simulink model "demo3c"  (Simulink 7.4)
settings: Solver=ode3  StartTime=0.0  StopTime=4  MinStep=0.000  RelTol=1e-3
undefined symbols (not defined in the file): disturb, fgamma, lambda11, lambda12, lambda21, lambda22, Mdisturb
libraries: roblocks x3, simulink x1
settings Model: Creator=pic  LastModifiedBy=acolome  ExtModeTrigMode=oneshot  ExtModeArmWhenConnect=off
settings DataIOCC: LimitDataPoints=off
settings OptimizationCC: BlockReduction=off  BooleanDataType=off  InitFltsAndDblsToZero=on
settings DebuggingCC: SaveWithParameterizedLinksMsg=none  SignalResolutionControl=TryResolveAllWithWarning  SolverPrmCheckMsg=none  MultiTaskDSMMsg=warning  MultiTaskCondExecSysMsg=none  StrictBusMsg=None
settings HardwareCC: TargetUnknown=on
settings RTWCC: IncludeERTFirstTime=on
settings GRTTargetCC: ModelReferenceCompliant=off  ParMdlRefBuildCompliant=off  CompOptLevelCompliant=off  MatFileLogging=off

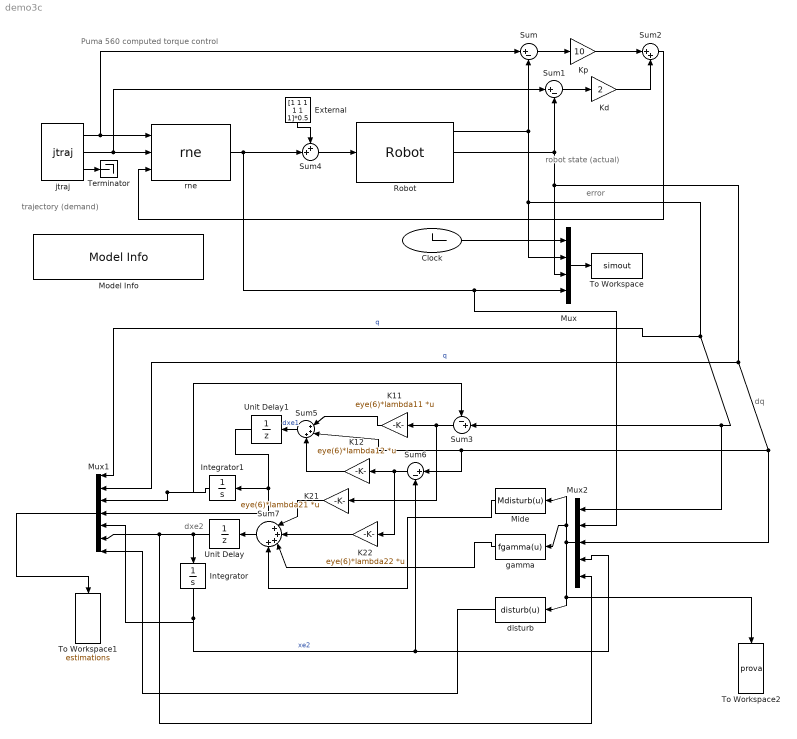
== system demo3c ==
  note: Puma 560 computed torque control
  note: trajectory
      | (demand)
  note: robot state
      | (actual)
  note: error
  note: dq
  note: dxe2
  Clock : Clock
      settings: Decimation=100
  External : Constant  Value=[1 1 1 1 1 1]*0.5  OutDataType=fixdt(1, 16)  OutScaling=2^0
  Integrator : Integrator
  Integrator1 : Integrator
  K11 : Gain  Gain=eye(6)*lambda11  Multiplication=Matrix(K*u)  ParameterDataType=fixdt(1, 16)  ParameterScaling=2^0  OutDataType=fixdt(1, 16)  OutScaling=2^0
  K12 : Gain  Gain=eye(6)*lambda12  Multiplication=Matrix(K*u)  ParameterDataType=fixdt(1, 16)  ParameterScaling=2^0  OutDataType=fixdt(1, 16)  OutScaling=2^0
  K21 : Gain  Gain=eye(6)*lambda21  Multiplication=Matrix(K*u)  ParameterDataType=fixdt(1, 16)  ParameterScaling=2^0  OutDataType=fixdt(1, 16)  OutScaling=2^0
  K22 : Gain  Gain=eye(6)*lambda22  Multiplication=Matrix(K*u)  ParameterDataType=fixdt(1, 16)  ParameterScaling=2^0  OutDataType=fixdt(1, 16)  OutScaling=2^0
  Kd : Gain  Gain=2  SaturateOnIntegerOverflow=on  OutDataTypeStr=Inherit: Same as input  ParamDataTypeStr=Inherit: Same as input
  Kp : Gain  Gain=10  SaturateOnIntegerOverflow=on  OutDataTypeStr=Inherit: Same as input  ParamDataTypeStr=Inherit: Same as input
  Mide : MATLABFcn  MATLABFcn=Mdisturb(u)
  Model Info : simulink/Model-Wide Utilities/Model Info  SystemSampleTime=-1  InitialBlockCM=none  BlockCM=none  Frame=on  DisplayStringWithTags=|  HorizontalTextAlignment=Left  LeftAlignmentValue=0.02  SourceBlockDiagram=demo3c  TagMaxNumber=20
      | Puma560 computed torque control
      | %<Creator>
      | %<LastModificationDate>
  Mux : Mux
  Mux1 : Mux  Inputs=7
  Mux2 : Mux  Inputs=5
  Robot : roblocks/Robot  SystemSampleTime=-1  robot=p560  q0=[0 0 0 0 0 0]
  Sum : Sum  Inputs=|+-  SaturateOnIntegerOverflow=on  InputSameDT=on  OutDataTypeStr=Inherit: Same as first input
  Sum1 : Sum  Inputs=|+-  SaturateOnIntegerOverflow=on  InputSameDT=on  OutDataTypeStr=Inherit: Same as first input
  Sum2 : Sum  Inputs=|++  SaturateOnIntegerOverflow=on  InputSameDT=on  OutDataTypeStr=Inherit: Same as first input
  Sum3 : Sum  Inputs=-+|  OutDataType=fixdt(1, 16)  OutScaling=2^0
  Sum4 : Sum  Inputs=++|  OutDataType=fixdt(1, 16)  OutScaling=2^0
  Sum5 : Sum  Inputs=|+++  OutDataType=fixdt(1, 16)  OutScaling=2^0
  Sum6 : Sum  Inputs=|+-  OutDataType=fixdt(1, 16)  OutScaling=2^0
  Sum7 : Sum  Inputs=|++++  OutDataType=fixdt(1, 16)  OutScaling=2^0
  Terminator : Terminator
  To Workspace : ToWorkspace  VariableName=simout  SampleTime=-1  SaveFormat=Array
  To Workspace1 : ToWorkspace  VariableName=estimations  SampleTime=-1  SaveFormat=Array
  To Workspace2 : ToWorkspace  VariableName=prova  SampleTime=-1  SaveFormat=Array
  Unit Delay : UnitDelay  SampleTime=-1
  Unit Delay1 : UnitDelay  SampleTime=-1
  disturb : MATLABFcn  MATLABFcn=disturb(u)
  gamma : MATLABFcn  MATLABFcn=fgamma(u)
  jtraj : roblocks/jtraj  SystemSampleTime=-1  q0=[pi/4 pi/2 -pi/2 0 0 0]  qf=[pi/4 pi/2 -pi/2 0 0 0]  tmax=4
      link override MATLAB Fcn: MATLABFcn=squeeze(interp1(t,q,u))
      link override MATLAB Fcn1: MATLABFcn=squeeze(interp1(t,qd,u))
      link override MATLAB Fcn2: MATLABFcn=squeeze(interp1(t,qdd,u))
  rne : roblocks/rne  SystemSampleTime=-1  robot=p560  grav=[0 0 9.81]
  wires:
  Sum/1 -> Kp/1
  Kp/1 -> Sum2/1
  Robot/1 -> Sum/2, Mux/2, Mux1/1, Sum3/2, Mux2/1  "q"
  Robot/2 -> Sum1/2, Mux/3, Sum5/2, Sum6/1, Mux2/3, Mux1/2  "q"
  Sum2/1 -> rne/3
  rne/1 -> Sum4/2, Mux/4, Mux2/2
  jtraj/1 -> Sum/1, rne/1
  jtraj/2 -> rne/2, Sum1/1
  Mux/1 -> To Workspace/1
  Clock/1 -> Mux/1
  Sum1/1 -> Kd/1
  Kd/1 -> Sum2/2
  jtraj/3 -> Terminator/1
  Sum4/1 -> Robot/1
  External/1 -> Sum4/1
  K11/1 -> Sum5/1
  Sum3/1 -> K11/1, K21/1
  Sum6/1 -> K12/1, K22/1
  K12/1 -> Sum5/3
  K22/1 -> Sum7/2
  K21/1 -> Sum7/1
  Mux1/1 -> To Workspace1/1
  Integrator1/1 -> Mux1/3, Sum3/1
  Integrator/1 -> Mux1/5, Sum6/2, Mux2/4  "xe2"
  gamma/1 -> Sum7/3
  Mide/1 -> Sum7/4
  disturb/1 -> Mux1/7
  Mux2/1 -> gamma/1, Mide/1, disturb/1, To Workspace2/1
  Sum7/1 -> Unit Delay/1
  Unit Delay/1 -> Integrator/1, Mux1/6, Mux2/5
  Sum5/1 -> Unit Delay1/1  "dxe1"
  Unit Delay1/1 -> Mux1/4, Integrator1/1
